simulink model "A5Q2a_PDG"  (R2018a)
settings: Solver=FixedStepDiscrete  StartTime=0.0  StopTime=15  FixedStep=0.001  RelTol=1e-3
libraries: simulink x1
settings Model: PauseTimes=30  Creator=jadm  LastModifiedBy=jadm

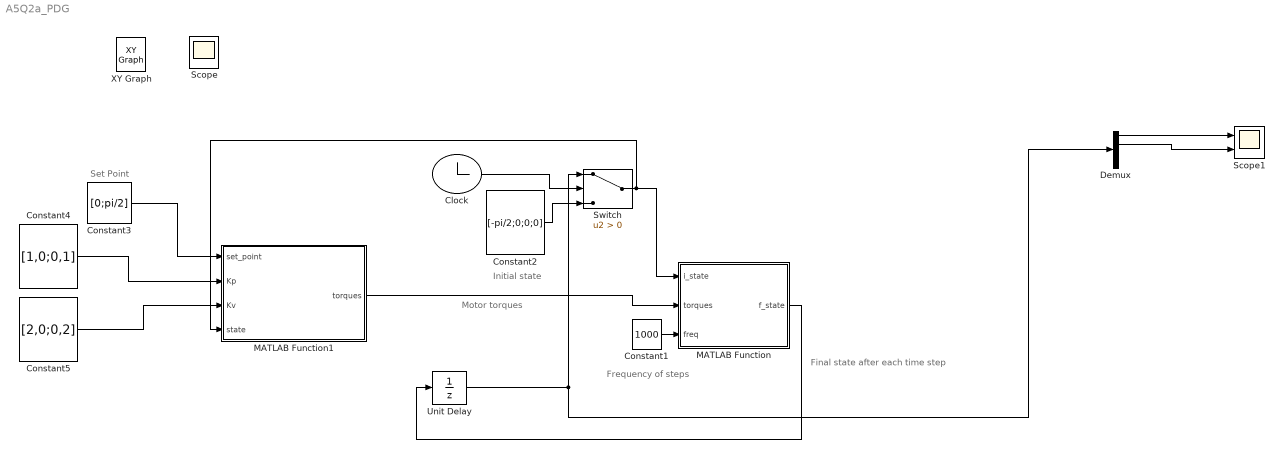
== system A5Q2a_PDG ==
  note: Motor torques
  note: Final state after each time step
  note: Initial state
  note: Frequency of steps
  note: Set Point
  Clock : Clock
  Constant1 : Constant  Value=1000  VectorParams1D=off
  Constant2 : Constant  Value=[-pi/2;0;0;0]  VectorParams1D=off
  Constant3 : Constant  Value=[0;pi/2]  VectorParams1D=off
  Constant4 : Constant  Value=[1,0;0,1]  VectorParams1D=off
  Constant5 : Constant  Value=[2,0;0,2]  VectorParams1D=off
  Demux : Demux
  MATLAB Function : MATLAB Function  TreatAsAtomicUnit=on
  MATLAB Function1 : MATLAB Function  TreatAsAtomicUnit=on
  Scope1 : Scope  NumInputPorts=2
  Switch : Switch  Criteria=u2 > Threshold
  Unit Delay : UnitDelay  SampleTime=-1
  Scope : Scope
  XY Graph : simulink/Sinks/XY Graph  IOType=viewer  xmin=-1  xmax=1  ymin=-1  ymax=1  st=-1
  wires:
  MATLAB Function1/1(torques) -> MATLAB Function/2(torques)
  Constant1/1 -> MATLAB Function/3(freq)
  Demux/1 -> Scope1/1
  Demux/2 -> Scope1/2
  Clock/1 -> Switch/2
  Constant2/1 -> Switch/3
  Switch/1 -> MATLAB Function1/4(state), MATLAB Function/1(i_state)
  MATLAB Function/1(f_state) -> Unit Delay/1
  Unit Delay/1 -> Demux/1, Switch/1
  Constant3/1 -> MATLAB Function1/1(set_point)
  Constant4/1 -> MATLAB Function1/2(Kp)
  Constant5/1 -> MATLAB Function1/3(Kv)

== matlab function A5Q2a_PDG/MATLAB Function1 ==
  data: set_point input; Kp input; Kv input; torques output; state input
function torques  = PDG_controller(set_point, Kp, Kv, state)
%given input set point and robot state output the desired torques based on
%the PD + G set point control method

%define values
L1 = 1; %m
L2 = 1; %m
m1 = 1; %kg
m2 = 1; %kg
g = 9.81; %m/s^2

%set q and qdot
q = state(1:2);
qdot = state(3:4);

%set up specfic angles
q1i = state(1);
q2i = state(2);

%set up G(q)
G = [((m1+m2)*g*L1*cos(q1i)+m2*g*L2*cos(q1i+q2i));(m2*g*L2*cos(q1i+q2i))];

torques = G + Kp*(set_point - q) - Kv*qdot;

== matlab function A5Q2a_PDG/MATLAB Function ==
  data: i_state input; f_state output; torques input; freq input
function f_state  = Robot(i_state, torques, freq)
%Given the initial state and motor torques for the manipulator in Ch.6,
%p.87 of the notes, compute the final state

%define values
L1 = 1; %m
L2 = 1; %m
m1 = 1; %kg
m2 = 1; %kg
g = 9.81; %m/s^2

%set up angle array
q1i = i_state(1);
q2i = i_state(2);
q1doti = i_state(3);
q2doti = i_state(4);

%set up D,C and G matrices
D = [((m1+m2)*L1^2+m2*L2^2+2*m2*L1*L2*cos(q2i)),(m2*L2^2+m2*L1*L2*cos(q2i));...
    (m2*L2^2+m2*L1*L2*cos(q2i)),(m2*L2^2)];
C = [(-2*m2*L1*L2*(sin(q2i))*q2doti),(-1*m2*L1*L2*(sin(q2i))*q2doti);...
    (m2*L1*L2*(sin(q2i))*q1doti),0];
G = [((m1+m2)*g*L1*cos(q1i)+m2*g*L2*cos(q1i+q2i));(m2*g*L2*cos(q1i+q2i))];

%given inputs solve for initial angular acceleration of joints
accel = D\(torques - G - C*([q1doti;q2doti]));

q1dubdoti = accel(1);
q2dubdoti = accel(2);

% find next state given initial state using kinematics equations
q1f = q1i+(1/freq)*q1doti+0.5*(1/freq)^2*q1dubdoti;
q2f = q2i+(1/freq)*q2doti+0.5*(1/freq)^2*q2dubdoti;
q1dotf = q1doti+(1/freq)*q1dubdoti;
q2dotf = q2doti+(1/freq)*q2dubdoti;

f_state = [q1f;q2f;q1dotf;q2dotf];
